simulink model "TractorTrailerMathematicalModel"  (R2023b)
settings: Solver=VariableStepAuto  StartTime=0.0  StopTime=10.0  RelTol=1e-3
model mask{initialPosition=initialPosition, initialVelocity=initialVelocity, theta=theta, beta=beta}
  mask prompts: initialPosition "Initial Position:"; initialVelocity "Initial Velocity:"; theta "Trailer Orientation (rad) :"; beta "Tractor Orientation (rad) :"
model workspace (MAT data in the model file):
  beta = Simulink.Parameter
  beta.Value = 0
  beta.DataType = 'auto'
  beta.Complexity = 'real'
  beta.Dimensions = [1 1]
  initialPosition = Simulink.Parameter
  initialPosition.Value = [0 0 0]
  initialPosition.DataType = 'auto'
  initialPosition.Complexity = 'real'
  initialPosition.Dimensions = [1 3]
  initialVelocity = Simulink.Parameter
  initialVelocity.Value = [0 0 0]
  initialVelocity.DataType = 'auto'
  initialVelocity.Complexity = 'real'
  initialVelocity.Dimensions = [1 3]
  theta = Simulink.Parameter
  theta.Value = 0
  theta.DataType = 'auto'
  theta.Complexity = 'real'
  theta.Dimensions = [1 1]
undefined symbols (not defined in the file): tractor, vehicleDimension
settings Model: ParameterArgumentNames=beta,initialPosition,initialVelocity,theta  Creator=The MathWorks, Inc.  LastModifiedBy=The MathWorks, Inc.
settings OptimizationCC: ReuseModelBlockBuffer=off

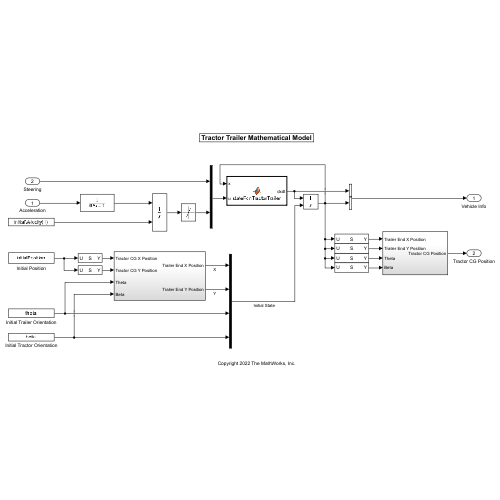
[thumbnail: Simulink's stored preview of the top-level diagram]
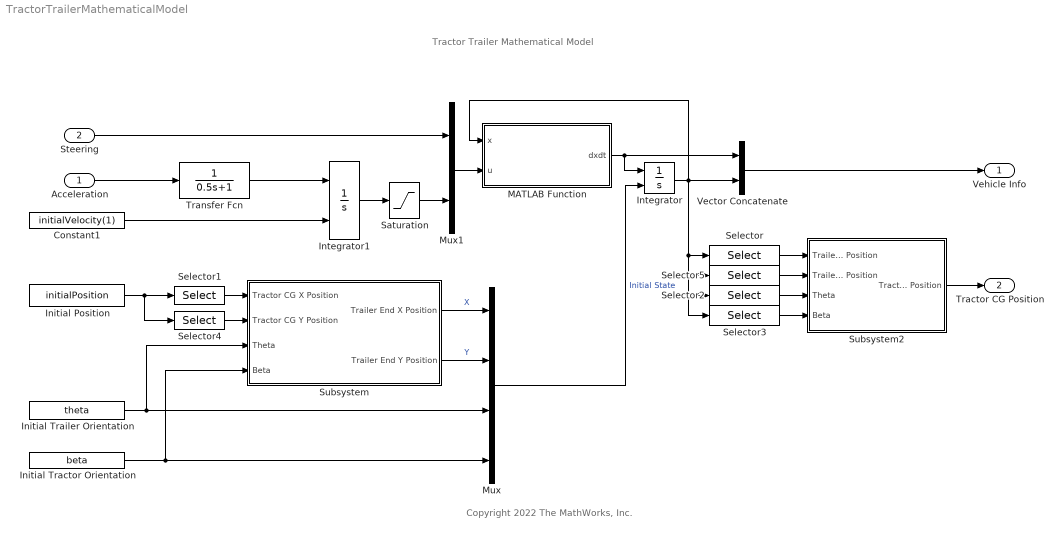
== system TractorTrailerMathematicalModel ==
  note: Copyright 2022 The MathWorks, Inc.
  note: Tractor Trailer Mathematical Model
  Acceleration : Inport
  Steering : Inport  Port=2
  Constant1 : Constant  Value=initialVelocity(1)
  Initial Position : Constant  Value=initialPosition
  Initial Tractor Orientation : Constant  Value=beta
  Initial Trailer Orientation : Constant  Value=theta
  Integrator : Integrator  InitialConditionSource=external
  Integrator1 : Integrator  InitialConditionSource=external
  MATLAB Function : MATLAB Function  TreatAsAtomicUnit=on
  Mux : Mux
  Mux1 : Mux  Inputs=2
  Saturation : Saturate  UpperLimit=30  LowerLimit=0
  Selector : Selector  InputPortWidth=4  IndexOptions=Index vector (dialog)  Indices=1  OutputSizes=1
  Selector1 : Selector  InputPortWidth=3  IndexOptions=Index vector (dialog)  Indices=1  OutputSizes=1
  Selector2 : Selector  InputPortWidth=4  IndexOptions=Index vector (dialog)  Indices=3  OutputSizes=1
  Selector3 : Selector  InputPortWidth=4  IndexOptions=Index vector (dialog)  Indices=4  OutputSizes=1
  Selector4 : Selector  InputPortWidth=3  IndexOptions=Index vector (dialog)  Indices=2  OutputSizes=1
  Selector5 : Selector  InputPortWidth=4  IndexOptions=Index vector (dialog)  Indices=2  OutputSizes=1
  Subsystem : Subsystem
  Subsystem2 : Subsystem
  Transfer Fcn : TransferFcn  Denominator=[0.5 1]
  Vector Concatenate : Concatenate
  Vehicle Info : Outport
  Tractor CG Position : Outport  Port=2
  wires:
  Acceleration/1 -> Transfer Fcn/1
  Integrator1/1 -> Saturation/1
  Constant1/1 -> Integrator1/2
  Transfer Fcn/1 -> Integrator1/1
  Steering/1 -> Mux1/1
  Saturation/1 -> Mux1/2
  MATLAB Function/1(dxdt) -> Integrator/1, Vector Concatenate/1
  Vector Concatenate/1 -> Vehicle Info/1
  Initial Tractor Orientation/1 -> Mux/4, Subsystem/4(Beta)
  Initial Trailer Orientation/1 -> Mux/3, Subsystem/3(Theta)
  Mux/1 -> Integrator/2  "Initial State"
  Selector/1 -> Subsystem2/1(Trailer End X Position)
  Selector2/1 -> Subsystem2/3(Theta)
  Integrator/1 -> Selector5/1, Selector2/1, Selector3/1, Selector/1, MATLAB Function/1(x), Vector Concatenate/2
  Selector3/1 -> Subsystem2/4(Beta)
  Subsystem2/1(Tractor CG Position) -> Tractor CG Position/1
  Subsystem/1(Trailer End X Position) -> Mux/1  "X"
  Subsystem/2(Trailer End Y Position) -> Mux/2  "Y"
  Selector1/1 -> Subsystem/1(Tractor CG X Position)
  Initial Position/1 -> Selector4/1, Selector1/1
  Selector4/1 -> Subsystem/2(Tractor CG Y Position)
  Selector5/1 -> Subsystem2/2(Trailer End Y Position)
  Mux1/1 -> MATLAB Function/2(u)

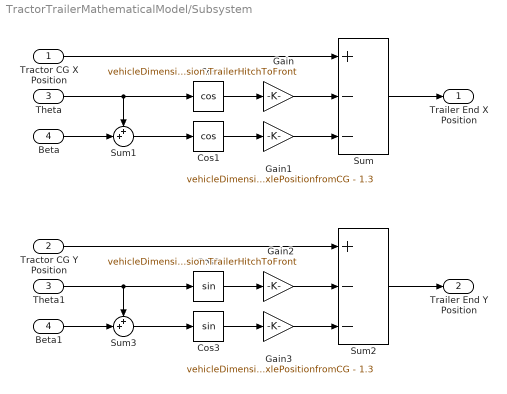
== system TractorTrailerMathematicalModel/Subsystem ==
  Tractor CG X Position : Inport
  Tractor CG Y Position : Inport  Port=2
  Theta : Inport  Port=3
  Beta : Inport  Port=4
  Beta1 : InportShadow  Port=4
  Cos : Trigonometry  Operator=cos
  Cos1 : Trigonometry  Operator=cos
  Cos2 : Trigonometry
  Cos3 : Trigonometry
  Gain : Gain  Gain=vehicleDimension.TrailerLength - vehicleDimension.TrailerHitchToFront
  Gain1 : Gain  Gain=vehicleDimension.InterConnection + vehicleDimension.TractorLength - vehicleDimension.TractorEndToHitch - tractor.FrontAxlePositionfromCG - 1.3
  Gain2 : Gain  Gain=vehicleDimension.TrailerLength - vehicleDimension.TrailerHitchToFront
  Gain3 : Gain  Gain=vehicleDimension.InterConnection + vehicleDimension.TractorLength - vehicleDimension.TractorEndToHitch - tractor.FrontAxlePositionfromCG - 1.3
  Sum : Sum  Inputs=+--
  Sum1 : Sum  Inputs=++|
  Sum2 : Sum  Inputs=+--
  Sum3 : Sum  Inputs=++|
  Theta1 : InportShadow  Port=3
  Trailer End X Position : Outport
  Trailer End Y Position : Outport  Port=2
  wires:
  Theta/1 -> Sum1/1, Cos/1
  Cos/1 -> Gain/1
  Gain/1 -> Sum/2
  Gain1/1 -> Sum/3
  Cos1/1 -> Gain1/1
  Sum/1 -> Trailer End X Position/1
  Tractor CG X Position/1 -> Sum/1
  Beta/1 -> Sum1/2
  Sum1/1 -> Cos1/1
  Tractor CG Y Position/1 -> Sum2/1
  Sum2/1 -> Trailer End Y Position/1
  Theta1/1 -> Cos2/1, Sum3/1
  Gain2/1 -> Sum2/2
  Gain3/1 -> Sum2/3
  Cos3/1 -> Gain3/1
  Cos2/1 -> Gain2/1
  Beta1/1 -> Sum3/2
  Sum3/1 -> Cos3/1

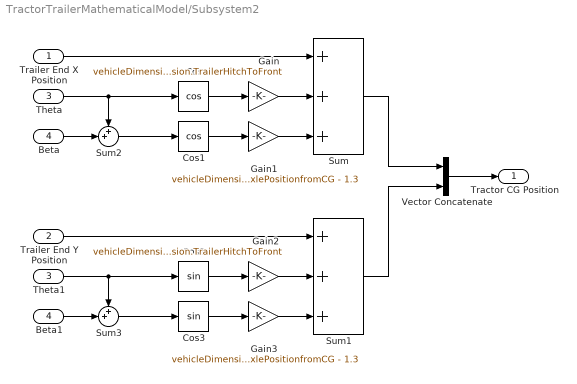
== system TractorTrailerMathematicalModel/Subsystem2 ==
  Trailer End X Position : Inport
  Trailer End Y Position : Inport  Port=2
  Theta : Inport  Port=3
  Beta : Inport  Port=4
  Beta1 : InportShadow  Port=4
  Cos : Trigonometry  Operator=cos
  Cos1 : Trigonometry  Operator=cos
  Cos2 : Trigonometry
  Cos3 : Trigonometry
  Gain : Gain  Gain=vehicleDimension.TrailerLength - vehicleDimension.TrailerHitchToFront
  Gain1 : Gain  Gain=vehicleDimension.InterConnection + vehicleDimension.TractorLength - vehicleDimension.TractorEndToHitch - tractor.FrontAxlePositionfromCG - 1.3
  Gain2 : Gain  Gain=vehicleDimension.TrailerLength - vehicleDimension.TrailerHitchToFront
  Gain3 : Gain  Gain=vehicleDimension.InterConnection + vehicleDimension.TractorLength - vehicleDimension.TractorEndToHitch - tractor.FrontAxlePositionfromCG - 1.3
  Sum : Sum  Inputs=+++
  Sum1 : Sum  Inputs=+++
  Sum2 : Sum  Inputs=++|
  Sum3 : Sum  Inputs=++|
  Theta1 : InportShadow  Port=3
  Vector Concatenate : Concatenate
  Tractor CG Position : Outport
  wires:
  Theta/1 -> Sum2/1, Cos/1
  Cos/1 -> Gain/1
  Gain/1 -> Sum/2
  Gain1/1 -> Sum/3
  Cos1/1 -> Gain1/1
  Sum/1 -> Vector Concatenate/1
  Trailer End X Position/1 -> Sum/1
  Trailer End Y Position/1 -> Sum1/1
  Cos2/1 -> Gain2/1
  Theta1/1 -> Sum3/1, Cos2/1
  Gain3/1 -> Sum1/3
  Cos3/1 -> Gain3/1
  Gain2/1 -> Sum1/2
  Beta1/1 -> Sum3/2
  Sum3/1 -> Cos3/1
  Beta/1 -> Sum2/2
  Sum2/1 -> Cos1/1
  Vector Concatenate/1 -> Tractor CG Position/1
  Sum1/1 -> Vector Concatenate/2

== matlab function TractorTrailerMathematicalModel/MATLAB Function ==
  data: x input; u input; dxdt output; vehicleDimension parameter
function dxdt = stateFcnTractorTrailer(x,u,vehicleDimension)%#codegen
dxdt = zeros(4,1);
dxdt = helperStateFcnTractorTrailer(x, u, vehicleDimension.TractorLength - vehicleDimension.TractorEndToHitch , vehicleDimension.TrailerLength - vehicleDimension.TrailerHitchToFront, vehicleDimension.InterConnection);
